simulink model "problem1Simplified"  (R2014a)
settings: Solver=ode45  StartTime=0.0  StopTime=20.0  RelTol=1e-3
undefined symbols (not defined in the file or in its folder): den1, den2, num1, num2
settings Model: Creator=cunnia3  LastModifiedBy=cunnia3

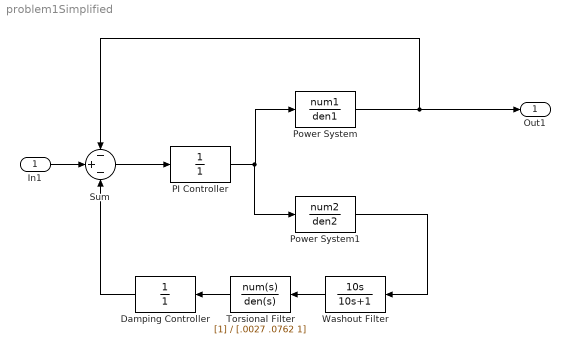
== system problem1Simplified ==
  In1 : Inport
  Damping Controller : TransferFcn  Denominator=[1]
  PI Controller : TransferFcn  Denominator=[1]
  Power System : TransferFcn  Numerator=num1  Denominator=den1
  Power System1 : TransferFcn  Numerator=num2  Denominator=den2
  Sum : Sum  Inputs=-+-
  Torsional Filter : TransferFcn  Denominator=[.0027 .0762 1]
  Washout Filter : TransferFcn  Numerator=[10 0]  Denominator=[10 1]
  Out1 : Outport
  wires:
  PI Controller/1 -> Power System1/1, Power System/1
  Sum/1 -> PI Controller/1
  Washout Filter/1 -> Torsional Filter/1
  Power System/1 -> Out1/1, Sum/1
  Torsional Filter/1 -> Damping Controller/1
  In1/1 -> Sum/2
  Damping Controller/1 -> Sum/3
  Power System1/1 -> Washout Filter/1
